simulink model "Chlorhexidine_Removal_System"  (R2024b)
settings: Solver=VariableStepAuto  StartTime=0.0  StopTime=10.0  RelTol=1e-3
settings Model: Creator=jakeo  LastModifiedBy=jakeo

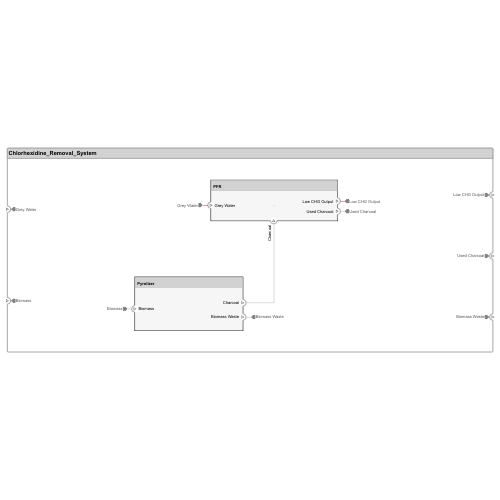
[thumbnail: Simulink's stored preview of the top-level diagram]
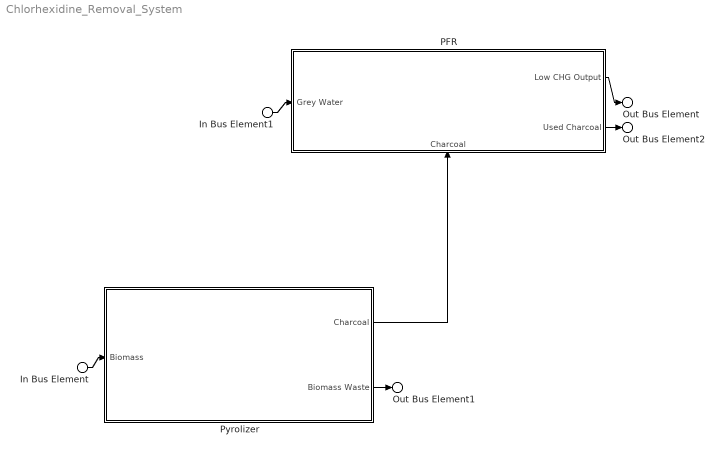
== system Chlorhexidine_Removal_System ==
  In Bus Element : Inport  PortName=Biomass
  In Bus Element1 : Inport  Port=2  PortName=Grey Water
  PFR : Subsystem
      settings: PortSchema="{\"entries\":[{\"content\":{\"headerSize\":26,\"margin\":15,\"minimumSpacing\":25,\"sides\":[{\"content\":{\"connectorIds\":[\"In2\"]},\"type\":\"ConnectorPlacement.EquallySpacedRectSide\",\"uuid\":\"fa1dbd3d-b57d-47b9-b4ef-0fe90e72294f\"},{\"content\":{\"connectorIds\":[\"Out1\",\"Out2\"],\"side\":\"RIGHT\"},\"type\":\"ConnectorPlacement.EquallySpacedRectSide\",\"uuid\":\"948d51fa-2dfa-4f43-89d3-5e64c8759b0a\"},{\"content\":{\"side\":\"TOP\"},\"type\":\"ConnectorPlacement.EquallySpacedRectSide\",\"uuid\":\"ae7cb2a6-ad1d-4ea0-b46a-3d468529a90e\"},{\"content\":{\"connectorIds\":[\"In1\"],\"side\":\"BOTTOM\"},\"type\":\"ConnectorPlacement.EquallySpacedRectSide\",\"uuid\":\"dc29dfe4-3980-46f5-bd0d-b60b93a30b71\"}]},\"type\":\"ConnectorPlacement.EquallySpacedConnector\",\"uuid\":\"9e4666f3-ab23-41a5-b5e5-84e2e52e58ec\"}],\"packageUris\":[\"http://schema.mathworks.com/mf0/Connector/R2020b\"],\"version\":\"1.0\"}"
  Pyrolizer : Subsystem
      settings: PortSchema="{\"entries\":[{\"content\":{\"headerSize\":26,\"margin\":15,\"minimumSpacing\":25,\"sides\":[{\"content\":{\"connectorIds\":[\"In1\"]},\"type\":\"ConnectorPlacement.EquallySpacedRectSide\",\"uuid\":\"fa1dbd3d-b57d-47b9-b4ef-0fe90e72294f\"},{\"content\":{\"connectorIds\":[\"Out1\",\"Out2\"],\"side\":\"RIGHT\"},\"type\":\"ConnectorPlacement.EquallySpacedRectSide\",\"uuid\":\"948d51fa-2dfa-4f43-89d3-5e64c8759b0a\"},{\"content\":{\"side\":\"TOP\"},\"type\":\"ConnectorPlacement.EquallySpacedRectSide\",\"uuid\":\"ae7cb2a6-ad1d-4ea0-b46a-3d468529a90e\"}]},\"type\":\"ConnectorPlacement.EquallySpacedConnector\",\"uuid\":\"9e4666f3-ab23-41a5-b5e5-84e2e52e58ec\"}],\"packageUris\":[\"http://schema.mathworks.com/mf0/Connector/R2020b\"],\"version\":\"1.0\"}"
  Out Bus Element : Outport  PortName=Low CHG Output
  Out Bus Element2 : Outport  Port=2  PortName=Used Charcoal
  Out Bus Element1 : Outport  Port=3  PortName=Biomass Waste
  wires:
  In Bus Element1/1 -> PFR/2(Grey Water)
  PFR/1(Low CHG Output) -> Out Bus Element/1
  In Bus Element/1 -> Pyrolizer/1(Biomass)
  Pyrolizer/1(Charcoal) -> PFR/1(Charcoal)
  Pyrolizer/2(Biomass Waste) -> Out Bus Element1/1
  PFR/2(Used Charcoal) -> Out Bus Element2/1

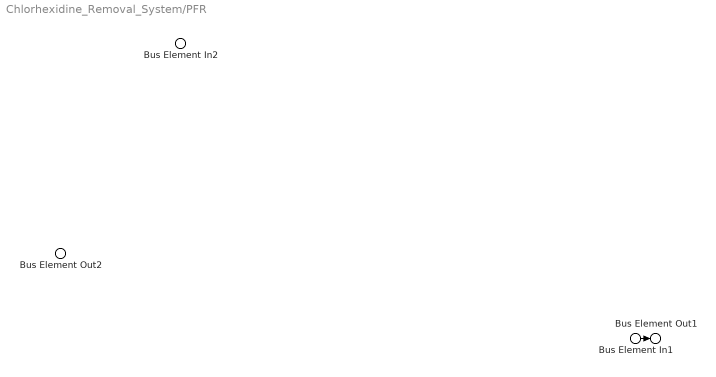
== system Chlorhexidine_Removal_System/PFR ==
  Bus Element In2 : Inport  PortName=Charcoal
  Bus Element In1 : Inport  Port=2  PortName=Grey Water
  Bus Element Out1 : Outport  PortName=Low CHG Output
  Bus Element Out2 : Outport  Port=2  PortName=Used Charcoal
  wires:
  Bus Element In1/1 -> Bus Element Out1/1

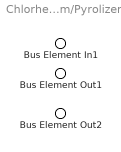
== system Chlorhexidine_Removal_System/Pyrolizer ==
  Bus Element In1 : Inport  PortName=Biomass
  Bus Element Out1 : Outport  PortName=Charcoal
  Bus Element Out2 : Outport  Port=2  PortName=Biomass Waste
